simulink model "chap02_100"  (R2020a)
settings: Solver=VariableStepAuto  StartTime=0.0  StopTime=10.0  RelTol=1e-3
settings Model: Creator=chen_w3  LastModifiedBy=chen_w3

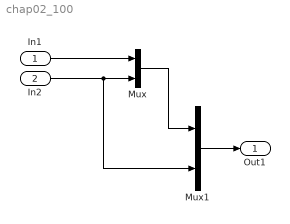
== system chap02_100 ==
  In1 : Inport
  In2 : Inport  Port=2
  Mux : Mux  Inputs=2
  Mux1 : Mux  Inputs=2
  Out1 : Outport
  wires:
  In1/1 -> Mux/1
  In2/1 -> Mux1/2, Mux/2
  Mux/1 -> Mux1/1
  Mux1/1 -> Out1/1
